simulink model "motorai"  (R2018b)
settings: Solver=FixedStepAuto  StartTime=0.0  StopTime=inf  FixedStep=SAMPLE_TIME  RelTol=1e-3
PreLoadFcn:
  | UserSettings
InitFcn:
  | ESTIMATION_SAMPLES = 50;
values from neighbouring files (symbols this model uses):
  ADC_bits = 12    [LQR_control_design.m]    (also in UserSettings.m)
  ADC_Vref = 3.3    [LQR_control_design.m]    (also in UserSettings.m)
  current_gain = 0.5    [LQR_control_design.m]    (also in UserSettings.m)
  current_offset = 1    [LQR_control_design.m]    (also in UserSettings.m)
  DATA_SAMPLING_FREQUENCY = 500    [UserSettings.m]
  K = -K    (= -0.383)    [LQG_control_design.m]    (also in LQR_control_design.m = -(1/R).*B'*Sinf; myLQR.m = -(1/R).*B'*Sinf; myREF.m = [Kw Ki])
  motorParameters = Parameters()    [UserSettings.m]
  omega_gain = 0.5    [LQR_control_design.m]    (also in UserSettings.m)
  omega_offset = 1    [LQR_control_design.m]    (also in UserSettings.m)
  PPR = 1000    [LQR_control_design.m]    (also in UserSettings.m)
  Q = 1/2*inv([(omega_max)^2 0 0; 0 (i_max)^2 0; 0 0 (int_max)^2])    [LQG_control_design.m]    (also in LQR_control_design.m = 1/2*inv([(omega_max)^2 0 ; 0 (i_max)^2]); myLQR.m = 1/2*inv([(omega_max)^2 0; 0 (i_max)^2]))
  R = inv([(v_max)^2])    [LQG_control_design.m]    (also in LQR_control_design.m; myLQR.m)
  SAMPLE_TIME = 5e-5    (= 5e-05)    [UserSettings.m]
  V_ACT = 12    [UserSettings.m]
  Vact = 12    [LQR_control_design.m]
undefined symbols (not defined in the file or in its folder): DiscIntNeverNeededParam
libraries: neural x275, mbedblockslib x7, fl_lib x5, nesl_utility x5, dspswit3 x3, elec_lib x3, powerlib_meascontrol x3, dspbuff3 x2, discretizing x1
(part 11 of 14)

== system motorai/Parameter Estimation & LQR /Function Fitting Neural Network1/Layer 2/Delays 1 ==
  "p{2}" : Inport  PortDimensions=166
      mask Display: e = 0.06;c1 = [120 230 180]/255;c2 = ([120 230 180]+0)/(256+128);c3 = ([120 230 180]+128)/(256+128);patch([0 1 1 0],[0 0 1 1],c1);patch([0 1 1 1-e 1-e 0+e],[0 0 1 1-e 0+e 0+e],c2);patch([0 0 1 1-e 0+e 0+e],[0 1 1 1-e 1-e 0+e],c3);plot([0 1 1 0 0],[0 0 1 1 0]);
  mux : Mux  Inputs=1
      mask Display: e = 0.06;c1 = [120 150 230]/255;c2 = ([120 150 230]+0)/383;c3 = ([120 150 230]+128)/383;patch([0 1 1 0],[0 0 1 1],c1);patch([0 1 1 1-e 1-e 0+e],[0 0 1 1-e 0+e 0+e],c2);patch([0 0 1 1-e 0+e 0+e],[0 1 1 1-e 1-e 0+e],c3);plot([0 1 1 0 0],[0 0 1 1 0]);disp('Mux')
  "pd{2,1}" : Outport
      mask Display: e = 0.06;c1 = [120 230 180]/255;c2 = ([120 230 180]+0)/(256+128);c3 = ([120 230 180]+128)/(256+128);patch([0 1 1 0],[0 0 1 1],c1);patch([0 1 1 1-e 1-e 0+e],[0 0 1 1-e 0+e 0+e],c2);patch([0 0 1 1-e 0+e 0+e],[0 1 1 1-e 1-e 0+e],c3);plot([0 1 1 0 0],[0 0 1 1 0]);
  wires:
  "p{2}"/1 -> mux/1
  mux/1 -> "pd{2,1}"/1
